simulink model "summary"  (R2022b)
settings: Solver=FixedStepAuto  StartTime=0.0  StopTime=20  FixedStep=0.1  RelTol=1e-3
values from neighbouring files (symbols this model uses):
  C_M = 1.1366    [MPC.m]
  C_T = 3.5611    [MPC.m]
  D_p = 0.1    [MPC.m]
  disturbance_f = 10    [MPC.m]    (also in generate_disturbance.m = f_min   + (f_max - f_min)   * rand(N, 1))
  disturbance_tau_x = 0.1    [MPC.m]    (also in generate_disturbance.m = tau_min + (tau_max - tau_min) * rand(N, 1))
  disturbance_tau_y = 0    [MPC.m]    (also in generate_disturbance.m = tau_min + (tau_max - tau_min) * rand(N, 1))
  disturbance_tau_z = 0    [MPC.m]    (also in generate_disturbance.m = tau_min + (tau_max - tau_min) * rand(N, 1))
  f_max = 10    [MPC.m]    (also in generate_disturbance.m)
  ModelInit_Att_x = 0    [MPC.m]
  ModelInit_Att_y = 0    [MPC.m]
  ModelInit_Att_z = 0    [MPC.m]
  ModelInit_Pos_x = 0    [MPC.m]
  ModelInit_Pos_y = 0    [MPC.m]
  ModelInit_Pos_z = 0    [MPC.m]
  ModelParam_c_M = 1.779e-07*2    (= 3.558e-07)    [MPC.m]
  ModelParam_c_T = 1.105e-05    [MPC.m]
  ModelParam_d = 0.225    [MPC.m]
  ModelParam_g = 9.8    [MPC.m]
  ModelParam_I_xx = 0.0211    [MPC.m]
  ModelParam_I_yy = 0.0219    [MPC.m]
  ModelParam_I_zz = 0.0366    [MPC.m]
  ModelParam_J_RP = 0.0001287    [MPC.m]
  ModelParam_m = 1.4    [MPC.m]
  p = 1.225    [MPC.m]    (also in draw_real_and_posiblility.m = alpha_smooth * p + (1 - alpha_smooth) * p_prev)
  tau_max = 0.1    [MPC.m]    (also in generate_disturbance.m = 0.25)
libraries: mpclib x3
settings Model: Creator=12854  LastModifiedBy=12854
settings OptimizationCC: BlockReduction=off  DefaultParameterBehavior=Inlined  BufferReuse=off

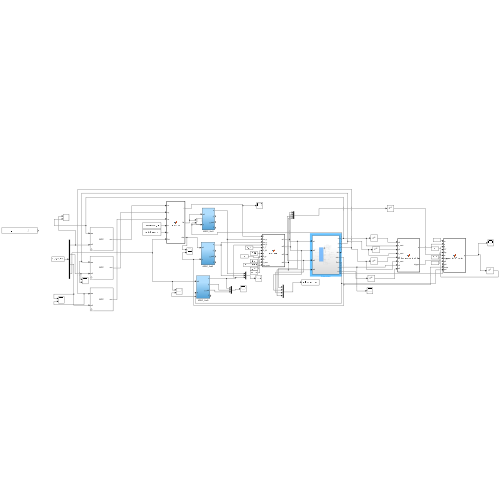
[thumbnail: Simulink's stored preview of the top-level diagram]
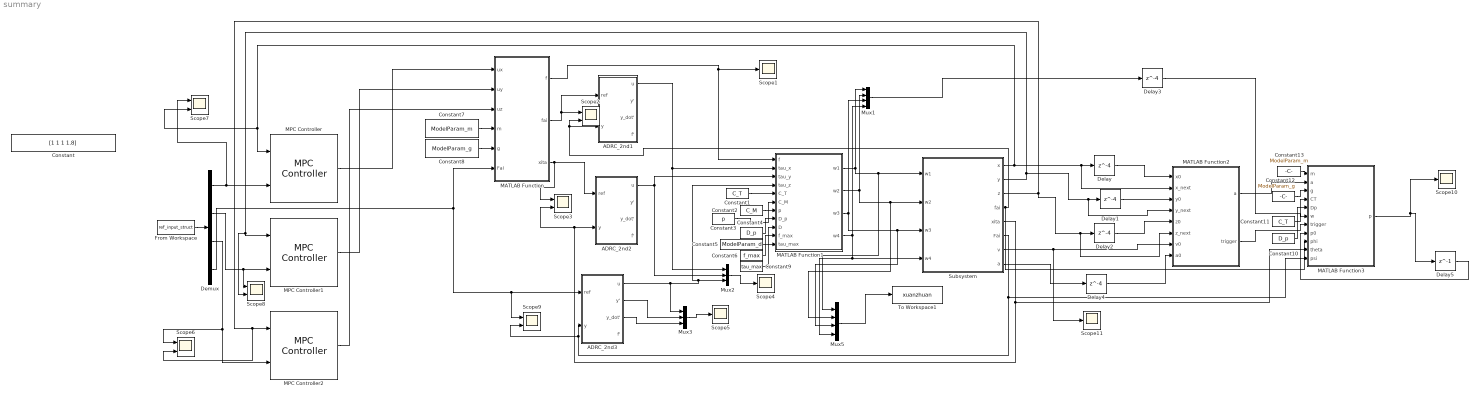
== system summary ==
  ADRC_2nd1 : Subsystem
  ADRC_2nd2 : Subsystem
  ADRC_2nd3 : Subsystem
  Constant : Constant  Value=[1 1 1 1.8]
  Constant1 : Constant  Value=C_T
  Constant10 : Constant  Value=D_p
  Constant11 : Constant  Value=C_T
  Constant12 : Constant  Value=ModelParam_g
  Constant13 : Constant  Value=ModelParam_m
  Constant2 : Constant  Value=C_M
  Constant3 : Constant  Value=p
  Constant4 : Constant  Value=D_p
  Constant5 : Constant  Value=ModelParam_d
  Constant6 : Constant  Value=f_max
  Constant7 : Constant  Value=ModelParam_m
  Constant8 : Constant  Value=ModelParam_g
  Constant9 : Constant  Value=tau_max
  Delay{,1..4} (5 alike) : Delay  DelayLength=4  InitialCondition=0
  Delay5 : Delay  DelayLength=1  InitialCondition=1.225
  Demux : Demux
  From Workspace : FromWorkspace  VariableName=ref_input_struct
  MATLAB Function : MATLAB Function  TreatAsAtomicUnit=on
  MATLAB Function1 : MATLAB Function  TreatAsAtomicUnit=on
  MATLAB Function2 : MATLAB Function  TreatAsAtomicUnit=on
  MATLAB Function3 : MATLAB Function  TreatAsAtomicUnit=on
  MPC Controller : mpclib/MPC Controller  SCDEnableBlockLinearizationSpecification=on  mpcobj=mpcobj_x  x0=[]  is_multiple=0  enable_value=0  return_u0=off  updateMPCinCallerWorkspace=on  md_inport=off  mv_inport=off  uref_inport=off  return_cost=off  return_mvseq=off  return_qpstatus=off  return_xseq=off  return_state=off  return_ovseq=off  state_inport=off  umin_inport=off  umax_inport=off  ymin_inport=off  ymax_inport=off  cc_inport=off  ywt_inport=off  uwt_inport=off  duwt_inport=off  rhoeps_inport=off  pm_inport=off  MaximumP=10  HorizonChoice=FixedHorizon  n_ts=0.1  n_p=10  n_mv=1  n_md=0  n_ud=0  n_mo=1  n_uo=0  BlockDataType=double  SampleTimeInherited=off  switch_inport=off
  MPC Controller1 : mpclib/MPC Controller  SCDEnableBlockLinearizationSpecification=on  mpcobj=mpcobj_y  x0=[]  is_multiple=0  enable_value=0  return_u0=off  updateMPCinCallerWorkspace=on  md_inport=off  mv_inport=off  uref_inport=off  return_cost=off  return_mvseq=off  return_qpstatus=off  return_xseq=off  return_state=off  return_ovseq=off  state_inport=off  umin_inport=off  umax_inport=off  ymin_inport=off  ymax_inport=off  cc_inport=off  ywt_inport=off  uwt_inport=off  duwt_inport=off  rhoeps_inport=off  pm_inport=off  MaximumP=10  HorizonChoice=FixedHorizon  n_ts=0.1  n_p=10  n_mv=1  n_md=0  n_ud=0  n_mo=1  n_uo=0  BlockDataType=double  SampleTimeInherited=off  switch_inport=off
  MPC Controller2 : mpclib/MPC Controller  SCDEnableBlockLinearizationSpecification=on  mpcobj=mpcobj_z  x0=[]  is_multiple=0  enable_value=0  return_u0=off  updateMPCinCallerWorkspace=on  md_inport=off  mv_inport=off  uref_inport=off  return_cost=off  return_mvseq=off  return_qpstatus=off  return_xseq=off  return_state=off  return_ovseq=off  state_inport=off  umin_inport=off  umax_inport=off  ymin_inport=off  ymax_inport=off  cc_inport=off  ywt_inport=off  uwt_inport=off  duwt_inport=off  rhoeps_inport=off  pm_inport=off  MaximumP=10  HorizonChoice=FixedHorizon  n_ts=0.1  n_p=10  n_mv=1  n_md=0  n_ud=0  n_mo=1  n_uo=0  BlockDataType=double  SampleTimeInherited=off  switch_inport=off
  Mux1 : Mux
  Mux2 : Mux  Inputs=3
  Mux3 : Mux  Inputs=3
  Mux5 : Mux
  Scope{1,4..5,10..11} (5 alike) : Scope
  Scope{2..3,6..9} (6 alike) : Scope  NumInputPorts=2
  Subsystem : Subsystem
  To Workspace1 : ToWorkspace  VariableName=xuanzhuan  SaveFormat=Timeseries  SampleTime=-1
  wires:
  Subsystem/1(x) -> MPC Controller/1, Scope7/2, MATLAB Function2/2(x_next), Delay/1
  Subsystem/2(y) -> Scope8/2, MPC Controller1/1, MATLAB Function2/4(y_next), Delay1/1
  Subsystem/3(z) -> MATLAB Function2/6(z_next), Delay2/1, Scope6/2, MPC Controller2/1
  Demux/1 -> Scope7/1, MPC Controller/2
  Demux/2 -> Scope8/1, MPC Controller1/2
  Demux/3 -> Scope6/1, MPC Controller2/2
  From Workspace/1 -> Demux/1
  MPC Controller/1 -> MATLAB Function/1(ux)
  MPC Controller1/1 -> MATLAB Function/2(uy)
  MPC Controller2/1 -> MATLAB Function/3(uz)
  Demux/4 -> Scope9/1, ADRC_2nd3/1(ref), MATLAB Function/6(Fai)
  Constant8/1 -> MATLAB Function/5(g)
  Constant7/1 -> MATLAB Function/4(m)
  MATLAB Function/1(f) -> Scope1/1, MATLAB Function1/1(f)
  Subsystem/4(fai) -> ADRC_2nd1/2(y), Scope2/2, MATLAB Function3/9(phi)
  MATLAB Function/2(fai) -> ADRC_2nd1/1(ref), Scope2/1
  MATLAB Function/3(xita) -> ADRC_2nd2/1(ref), Scope3/1
  Subsystem/5(xita) -> MATLAB Function3/10(theta), ADRC_2nd2/2(y), Scope3/2
  Subsystem/6(Fai) -> MATLAB Function3/11(psi), Scope9/2, ADRC_2nd3/2(y)
  ADRC_2nd3/1(u) -> Mux2/3, MATLAB Function1/4(tau_z), Mux3/1
  MATLAB Function1/1(w1) -> Mux1/1, Mux5/1, Subsystem/1(w1)
  MATLAB Function1/2(w2) -> Mux1/2, Mux5/2, Subsystem/2(w2)
  MATLAB Function1/3(w3) -> Mux1/3, Mux5/3, Subsystem/3(w3)
  MATLAB Function1/4(w4) -> Subsystem/4(w4), Mux5/4, Mux1/4
  Constant1/1 -> MATLAB Function1/5(C_T)
  Constant2/1 -> MATLAB Function1/6(C_M)
  Constant4/1 -> MATLAB Function1/8(D_p)
  Constant5/1 -> MATLAB Function1/9(D)
  Mux2/1 -> Scope4/1
  Constant6/1 -> MATLAB Function1/10(f_max)
  Constant9/1 -> MATLAB Function1/11(tau_max)
  Mux3/1 -> Scope5/1
  ADRC_2nd3/2(y') -> Mux3/2
  ADRC_2nd3/3(y_dot') -> Mux3/3
  ADRC_2nd1/1(u) -> Mux2/1, MATLAB Function1/2(tau_x)
  ADRC_2nd2/1(u) -> Mux2/2, MATLAB Function1/3(tau_y)
  Subsystem/7(v) -> Scope11/1, MATLAB Function2/7(v0)
  Delay/1 -> MATLAB Function2/1(x0)
  Delay1/1 -> MATLAB Function2/3(y0)
  Delay2/1 -> MATLAB Function2/5(z0)
  MATLAB Function2/1(a) -> MATLAB Function3/2(a)
  Constant10/1 -> MATLAB Function3/5(Dp)
  Constant11/1 -> MATLAB Function3/4(CT)
  Constant12/1 -> MATLAB Function3/3(g)
  Constant13/1 -> MATLAB Function3/1(m)
  Mux1/1 -> Delay3/1
  Delay3/1 -> MATLAB Function3/6(w)
  Subsystem/8(a) -> Delay4/1
  Delay4/1 -> MATLAB Function2/8(a0)
  MATLAB Function2/2(trigger) -> MATLAB Function3/7(trigger)
  Delay5/1 -> MATLAB Function3/8(p0)
  Constant3/1 -> MATLAB Function1/7(p)
  MATLAB Function3/1(p) -> Scope10/1, Delay5/1
  Mux5/1 -> To Workspace1/1

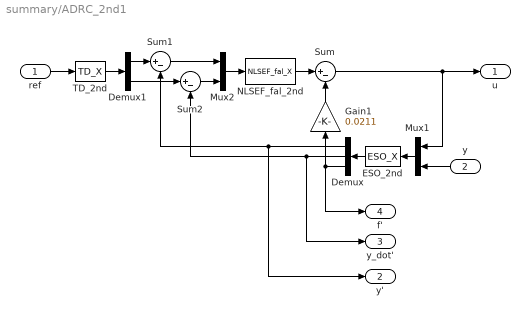
== system summary/ADRC_2nd1 ==
  ref : Inport
  y : Inport  Port=2
  Demux : Demux  Outputs=3
  Demux1 : Demux  Outputs=2
  ESO_2nd : S-Function  FunctionName=ESO_X  Parameters=CtrlParaX  SFunctionDeploymentMode=off  EnableBusSupport=off
  Gain1 : Gain  Gain=0.0211
  Mux1 : Mux  Inputs=2
  Mux2 : Mux  Inputs=2
  NLSEF_fal_2nd : S-Function  FunctionName=NLSEF_fal_X  Parameters=CtrlParaX  SFunctionDeploymentMode=off  EnableBusSupport=off
  Sum : Sum  Inputs=|+-
  Sum1 : Sum  Inputs=|+-
  Sum2 : Sum  Inputs=|+-
  TD_2nd : S-Function  FunctionName=TD_X  Parameters=CtrlParaX  SFunctionDeploymentMode=off  EnableBusSupport=off
  u : Outport  VectorParamsAs1DForOutWhenUnconnected=off
  y' : Outport  Port=2  VectorParamsAs1DForOutWhenUnconnected=off
  y_dot' : Outport  Port=3  VectorParamsAs1DForOutWhenUnconnected=off
  f' : Outport  Port=4  VectorParamsAs1DForOutWhenUnconnected=off
  wires:
  Mux2/1 -> NLSEF_fal_2nd/1
  ESO_2nd/1 -> Demux/1
  Demux1/2 -> Sum2/1
  ref/1 -> TD_2nd/1
  Demux/1 -> y'/1, Sum1/2
  TD_2nd/1 -> Demux1/1
  y/1 -> Mux1/2
  Gain1/1 -> Sum/2
  Demux/2 -> y_dot'/1, Sum2/2
  Demux1/1 -> Sum1/1
  Demux/3 -> Gain1/1, f'/1
  Sum2/1 -> Mux2/2
  Sum/1 -> Mux1/1, u/1
  NLSEF_fal_2nd/1 -> Sum/1
  Sum1/1 -> Mux2/1
  Mux1/1 -> ESO_2nd/1

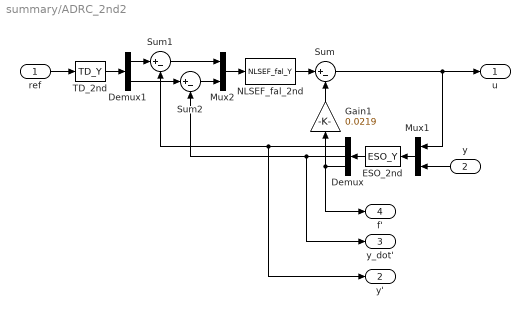
== system summary/ADRC_2nd2 ==
  ref : Inport
  y : Inport  Port=2
  Demux : Demux  Outputs=3
  Demux1 : Demux  Outputs=2
  ESO_2nd : S-Function  FunctionName=ESO_Y  Parameters=CtrlParaY  SFunctionDeploymentMode=off  EnableBusSupport=off
  Gain1 : Gain  Gain=0.0219
  Mux1 : Mux  Inputs=2
  Mux2 : Mux  Inputs=2
  NLSEF_fal_2nd : S-Function  FunctionName=NLSEF_fal_Y  Parameters=CtrlParaY  SFunctionDeploymentMode=off  EnableBusSupport=off
  Sum : Sum  Inputs=|+-
  Sum1 : Sum  Inputs=|+-
  Sum2 : Sum  Inputs=|+-
  TD_2nd : S-Function  FunctionName=TD_Y  Parameters=CtrlParaY  SFunctionDeploymentMode=off  EnableBusSupport=off
  u : Outport  VectorParamsAs1DForOutWhenUnconnected=off
  y' : Outport  Port=2  VectorParamsAs1DForOutWhenUnconnected=off
  y_dot' : Outport  Port=3  VectorParamsAs1DForOutWhenUnconnected=off
  f' : Outport  Port=4  VectorParamsAs1DForOutWhenUnconnected=off
  wires:
  Mux2/1 -> NLSEF_fal_2nd/1
  ESO_2nd/1 -> Demux/1
  Demux1/2 -> Sum2/1
  ref/1 -> TD_2nd/1
  Demux/1 -> y'/1, Sum1/2
  TD_2nd/1 -> Demux1/1
  y/1 -> Mux1/2
  Gain1/1 -> Sum/2
  Demux/2 -> y_dot'/1, Sum2/2
  Demux1/1 -> Sum1/1
  Demux/3 -> Gain1/1, f'/1
  Sum2/1 -> Mux2/2
  Sum/1 -> Mux1/1, u/1
  NLSEF_fal_2nd/1 -> Sum/1
  Sum1/1 -> Mux2/1
  Mux1/1 -> ESO_2nd/1

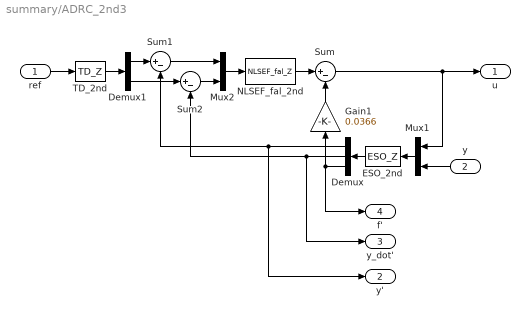
== system summary/ADRC_2nd3 ==
  ref : Inport
  y : Inport  Port=2
  Demux : Demux  Outputs=3
  Demux1 : Demux  Outputs=2
  ESO_2nd : S-Function  FunctionName=ESO_Z  Parameters=CtrlParaZ  SFunctionDeploymentMode=off  EnableBusSupport=off
  Gain1 : Gain  Gain=0.0366
  Mux1 : Mux  Inputs=2
  Mux2 : Mux  Inputs=2
  NLSEF_fal_2nd : S-Function  FunctionName=NLSEF_fal_Z  Parameters=CtrlParaZ  SFunctionDeploymentMode=off  EnableBusSupport=off
  Sum : Sum  Inputs=|+-
  Sum1 : Sum  Inputs=|+-
  Sum2 : Sum  Inputs=|+-
  TD_2nd : S-Function  FunctionName=TD_Z  Parameters=CtrlParaZ  SFunctionDeploymentMode=off  EnableBusSupport=off
  u : Outport  VectorParamsAs1DForOutWhenUnconnected=off
  y' : Outport  Port=2  VectorParamsAs1DForOutWhenUnconnected=off
  y_dot' : Outport  Port=3  VectorParamsAs1DForOutWhenUnconnected=off
  f' : Outport  Port=4  VectorParamsAs1DForOutWhenUnconnected=off
  wires:
  Mux2/1 -> NLSEF_fal_2nd/1
  ESO_2nd/1 -> Demux/1
  Demux1/2 -> Sum2/1
  ref/1 -> TD_2nd/1
  Demux/1 -> y'/1, Sum1/2
  TD_2nd/1 -> Demux1/1
  y/1 -> Mux1/2
  Gain1/1 -> Sum/2
  Demux/2 -> y_dot'/1, Sum2/2
  Demux1/1 -> Sum1/1
  Demux/3 -> Gain1/1, f'/1
  Sum2/1 -> Mux2/2
  Sum/1 -> Mux1/1, u/1
  NLSEF_fal_2nd/1 -> Sum/1
  Sum1/1 -> Mux2/1
  Mux1/1 -> ESO_2nd/1

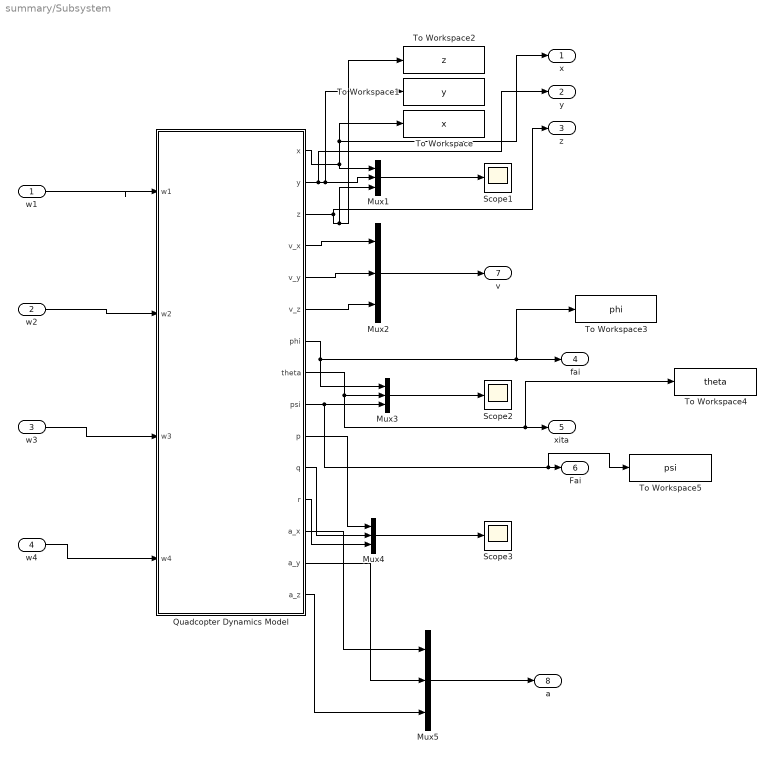
== system summary/Subsystem ==
  w1 : Inport
  w2 : Inport  Port=2
  w3 : Inport  Port=3
  w4 : Inport  Port=4
  Mux{1..5} (5 alike) : Mux  Inputs=3
  Quadcopter Dynamics Model : Subsystem
  Scope1 : Scope
  Scope2 : Scope
  Scope3 : Scope
  To Workspace : ToWorkspace  VariableName=x  SaveFormat=Timeseries  SampleTime=-1
  To Workspace1 : ToWorkspace  VariableName=y  SaveFormat=Timeseries  SampleTime=-1
  To Workspace2 : ToWorkspace  VariableName=z  SaveFormat=Timeseries  SampleTime=-1
  To Workspace3 : ToWorkspace  VariableName=phi  SaveFormat=Timeseries  SampleTime=-1
  To Workspace4 : ToWorkspace  VariableName=theta  SaveFormat=Timeseries  SampleTime=-1
  To Workspace5 : ToWorkspace  VariableName=psi  SaveFormat=Timeseries  SampleTime=-1
  x : Outport
  y : Outport  Port=2
  z : Outport  Port=3
  fai : Outport  Port=4
  xita : Outport  Port=5
  Fai : Outport  Port=6
  v : Outport  Port=7
  a : Outport  Port=8
  wires:
  Mux4/1 -> Scope3/1
  Mux3/1 -> Scope2/1
  Quadcopter Dynamics Model/2(y) -> y/1, To Workspace1/1, Mux1/2
  Quadcopter Dynamics Model/8(theta) -> To Workspace4/1, xita/1, Mux3/2
  Quadcopter Dynamics Model/5(v_y) -> Mux2/2
  Quadcopter Dynamics Model/1(x) -> x/1, To Workspace/1, Mux1/1
  Quadcopter Dynamics Model/6(v_z) -> Mux2/3
  Mux2/1 -> v/1
  Quadcopter Dynamics Model/12(r) -> Mux4/3
  Mux1/1 -> Scope1/1
  Quadcopter Dynamics Model/10(p) -> Mux4/1
  Quadcopter Dynamics Model/4(v_x) -> Mux2/1
  Quadcopter Dynamics Model/7(phi) -> Mux3/1, To Workspace3/1, fai/1
  Quadcopter Dynamics Model/3(z) -> To Workspace2/1, Mux1/3, z/1
  Quadcopter Dynamics Model/11(q) -> Mux4/2
  Quadcopter Dynamics Model/9(psi) -> To Workspace5/1, Fai/1, Mux3/3
  w1/1 -> Quadcopter Dynamics Model/1(w1)
  w2/1 -> Quadcopter Dynamics Model/2(w2)
  w3/1 -> Quadcopter Dynamics Model/3(w3)
  w4/1 -> Quadcopter Dynamics Model/4(w4)
  Quadcopter Dynamics Model/15(a_z) -> Mux5/3
  Quadcopter Dynamics Model/14(a_y) -> Mux5/2
  Quadcopter Dynamics Model/13(a_x) -> Mux5/1
  Mux5/1 -> a/1

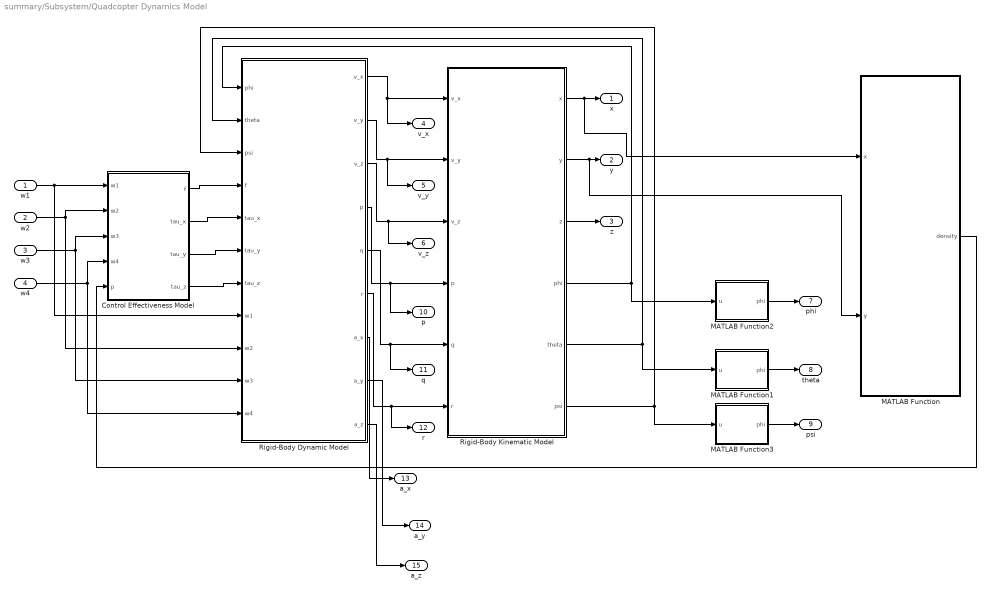
== system summary/Subsystem/Quadcopter Dynamics Model ==
  w1 : Inport
  w2 : Inport  Port=2
  w3 : Inport  Port=3
  w4 : Inport  Port=4
  Control Effectiveness Model : Subsystem
  MATLAB Function : MATLAB Function  TreatAsAtomicUnit=on
  MATLAB Function1 : MATLAB Function  TreatAsAtomicUnit=on
  MATLAB Function2 : MATLAB Function  TreatAsAtomicUnit=on
  MATLAB Function3 : MATLAB Function  TreatAsAtomicUnit=on
  Rigid-Body Dynamic Model : Subsystem
  Rigid-Body Kinematic Model : Subsystem
  x : Outport  VectorParamsAs1DForOutWhenUnconnected=off
  y : Outport  Port=2  VectorParamsAs1DForOutWhenUnconnected=off
  z : Outport  Port=3  VectorParamsAs1DForOutWhenUnconnected=off
  v_x : Outport  Port=4  VectorParamsAs1DForOutWhenUnconnected=off
  v_y : Outport  Port=5  VectorParamsAs1DForOutWhenUnconnected=off
  v_z : Outport  Port=6  VectorParamsAs1DForOutWhenUnconnected=off
  phi : Outport  Port=7  VectorParamsAs1DForOutWhenUnconnected=off
  theta : Outport  Port=8  VectorParamsAs1DForOutWhenUnconnected=off
  psi : Outport  Port=9  VectorParamsAs1DForOutWhenUnconnected=off
  p : Outport  Port=10  VectorParamsAs1DForOutWhenUnconnected=off
  q : Outport  Port=11  VectorParamsAs1DForOutWhenUnconnected=off
  r : Outport  Port=12  VectorParamsAs1DForOutWhenUnconnected=off
  a_x : Outport  Port=13  VectorParamsAs1DForOutWhenUnconnected=off
  a_y : Outport  Port=14  VectorParamsAs1DForOutWhenUnconnected=off
  a_z : Outport  Port=15  VectorParamsAs1DForOutWhenUnconnected=off
  wires:
  w1/1 -> Rigid-Body Dynamic Model/8(w1), Control Effectiveness Model/1(w1)
  Control Effectiveness Model/1(f) -> Rigid-Body Dynamic Model/4(f)
  w3/1 -> Rigid-Body Dynamic Model/10(w3), Control Effectiveness Model/3(w3)
  w4/1 -> Rigid-Body Dynamic Model/11(w4), Control Effectiveness Model/4(w4)
  w2/1 -> Rigid-Body Dynamic Model/9(w2), Control Effectiveness Model/2(w2)
  Rigid-Body Dynamic Model/4(p) -> Rigid-Body Kinematic Model/4(p), p/1
  Rigid-Body Dynamic Model/3(v_z) -> Rigid-Body Kinematic Model/3(v_z), v_z/1
  Rigid-Body Dynamic Model/6(r) -> Rigid-Body Kinematic Model/6(r), r/1
  Control Effectiveness Model/2(tau_x) -> Rigid-Body Dynamic Model/5(tau_x)
  Rigid-Body Dynamic Model/2(v_y) -> Rigid-Body Kinematic Model/2(v_y), v_y/1
  Rigid-Body Kinematic Model/1(x) -> MATLAB Function/1(x), x/1
  Rigid-Body Dynamic Model/5(q) -> Rigid-Body Kinematic Model/5(q), q/1
  Control Effectiveness Model/4(tau_z) -> Rigid-Body Dynamic Model/7(tau_z)
  Rigid-Body Kinematic Model/2(y) -> MATLAB Function/2(y), y/1
  Rigid-Body Kinematic Model/3(z) -> z/1
  Rigid-Body Dynamic Model/1(v_x) -> v_x/1, Rigid-Body Kinematic Model/1(v_x)
  Control Effectiveness Model/3(tau_y) -> Rigid-Body Dynamic Model/6(tau_y)
  Rigid-Body Kinematic Model/4(phi) -> MATLAB Function2/1(u), Rigid-Body Dynamic Model/1(phi)
  Rigid-Body Kinematic Model/5(theta) -> MATLAB Function1/1(u), Rigid-Body Dynamic Model/2(theta)
  Rigid-Body Kinematic Model/6(psi) -> MATLAB Function3/1(u), Rigid-Body Dynamic Model/3(psi)
  MATLAB Function2/1(phi) -> phi/1
  MATLAB Function1/1(phi) -> theta/1
  MATLAB Function3/1(phi) -> psi/1
  MATLAB Function/1(density) -> Control Effectiveness Model/5(p)
  Rigid-Body Dynamic Model/7(a_x) -> a_x/1
  Rigid-Body Dynamic Model/8(a_y) -> a_y/1
  Rigid-Body Dynamic Model/9(a_z) -> a_z/1

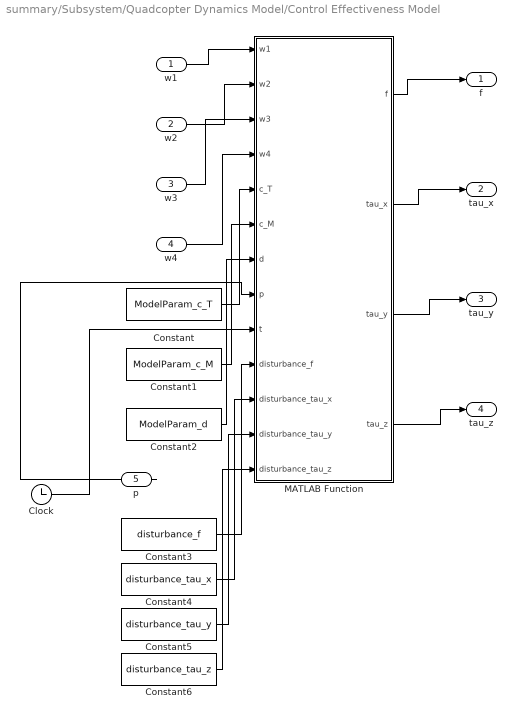
== system summary/Subsystem/Quadcopter Dynamics Model/Control Effectiveness Model ==
  w1 : Inport
  w2 : Inport  Port=2
  w3 : Inport  Port=3
  w4 : Inport  Port=4
  p : Inport  Port=5
  Clock : Clock
  Constant : Constant  Value=ModelParam_c_T
  Constant1 : Constant  Value=ModelParam_c_M
  Constant2 : Constant  Value=ModelParam_d
  Constant3 : Constant  Value=disturbance_f
  Constant4 : Constant  Value=disturbance_tau_x
  Constant5 : Constant  Value=disturbance_tau_y
  Constant6 : Constant  Value=disturbance_tau_z
  MATLAB Function : MATLAB Function  TreatAsAtomicUnit=on
  f : Outport  VectorParamsAs1DForOutWhenUnconnected=off
  tau_x : Outport  Port=2  VectorParamsAs1DForOutWhenUnconnected=off
  tau_y : Outport  Port=3  VectorParamsAs1DForOutWhenUnconnected=off
  tau_z : Outport  Port=4  VectorParamsAs1DForOutWhenUnconnected=off
  wires:
  Constant1/1 -> MATLAB Function/6(c_M)
  Constant/1 -> MATLAB Function/5(c_T)
  MATLAB Function/3(tau_y) -> tau_y/1
  MATLAB Function/1(f) -> f/1
  Constant2/1 -> MATLAB Function/7(d)
  MATLAB Function/4(tau_z) -> tau_z/1
  w3/1 -> MATLAB Function/3(w3)
  w1/1 -> MATLAB Function/1(w1)
  w4/1 -> MATLAB Function/4(w4)
  MATLAB Function/2(tau_x) -> tau_x/1
  w2/1 -> MATLAB Function/2(w2)
  p/1 -> MATLAB Function/8(p)
  Clock/1 -> MATLAB Function/9(t)
  Constant3/1 -> MATLAB Function/10(disturbance_f)
  Constant4/1 -> MATLAB Function/11(disturbance_tau_x)
  Constant5/1 -> MATLAB Function/12(disturbance_tau_y)
  Constant6/1 -> MATLAB Function/13(disturbance_tau_z)

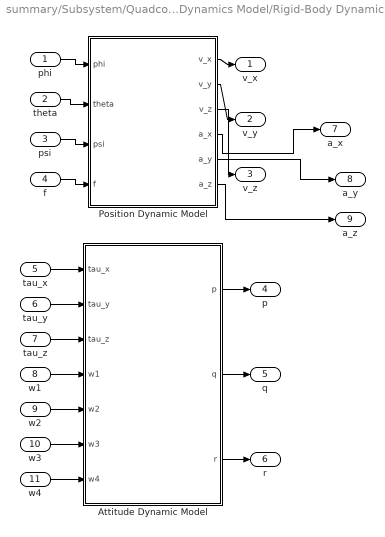
== system summary/Subsystem/Quadcopter Dynamics Model/Rigid-Body Dynamic Model ==
  phi : Inport
  theta : Inport  Port=2
  psi : Inport  Port=3
  f : Inport  Port=4
  tau_x : Inport  Port=5
  tau_y : Inport  Port=6
  tau_z : Inport  Port=7
  w1 : Inport  Port=8
  w2 : Inport  Port=9
  w3 : Inport  Port=10
  w4 : Inport  Port=11
  Attitude Dynamic Model : Subsystem
  Position Dynamic Model : Subsystem
  v_x : Outport  VectorParamsAs1DForOutWhenUnconnected=off
  v_y : Outport  Port=2  VectorParamsAs1DForOutWhenUnconnected=off
  v_z : Outport  Port=3  VectorParamsAs1DForOutWhenUnconnected=off
  p : Outport  Port=4  VectorParamsAs1DForOutWhenUnconnected=off
  q : Outport  Port=5  VectorParamsAs1DForOutWhenUnconnected=off
  r : Outport  Port=6  VectorParamsAs1DForOutWhenUnconnected=off
  a_x : Outport  Port=7  VectorParamsAs1DForOutWhenUnconnected=off
  a_y : Outport  Port=8  VectorParamsAs1DForOutWhenUnconnected=off
  a_z : Outport  Port=9  VectorParamsAs1DForOutWhenUnconnected=off
  wires:
  w3/1 -> Attitude Dynamic Model/6(w3)
  w1/1 -> Attitude Dynamic Model/4(w1)
  theta/1 -> Position Dynamic Model/2(theta)
  f/1 -> Position Dynamic Model/4(f)
  tau_x/1 -> Attitude Dynamic Model/1(tau_x)
  w2/1 -> Attitude Dynamic Model/5(w2)
  Attitude Dynamic Model/1(p) -> p/1
  w4/1 -> Attitude Dynamic Model/7(w4)
  Attitude Dynamic Model/2(q) -> q/1
  tau_y/1 -> Attitude Dynamic Model/2(tau_y)
  tau_z/1 -> Attitude Dynamic Model/3(tau_z)
  Position Dynamic Model/3(v_z) -> v_z/1
  Attitude Dynamic Model/3(r) -> r/1
  phi/1 -> Position Dynamic Model/1(phi)
  psi/1 -> Position Dynamic Model/3(psi)
  Position Dynamic Model/1(v_x) -> v_x/1
  Position Dynamic Model/2(v_y) -> v_y/1
  Position Dynamic Model/4(a_x) -> a_x/1
  Position Dynamic Model/5(a_y) -> a_y/1
  Position Dynamic Model/6(a_z) -> a_z/1

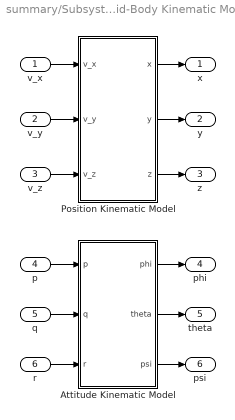
== system summary/Subsystem/Quadcopter Dynamics Model/Rigid-Body Kinematic Model ==
  v_x : Inport
  v_y : Inport  Port=2
  v_z : Inport  Port=3
  p : Inport  Port=4
  q : Inport  Port=5
  r : Inport  Port=6
  Attitude Kinematic Model : Subsystem
  Position Kinematic Model : Subsystem
  x : Outport  VectorParamsAs1DForOutWhenUnconnected=off
  y : Outport  Port=2  VectorParamsAs1DForOutWhenUnconnected=off
  z : Outport  Port=3  VectorParamsAs1DForOutWhenUnconnected=off
  phi : Outport  Port=4  VectorParamsAs1DForOutWhenUnconnected=off
  theta : Outport  Port=5  VectorParamsAs1DForOutWhenUnconnected=off
  psi : Outport  Port=6  VectorParamsAs1DForOutWhenUnconnected=off
  wires:
  v_x/1 -> Position Kinematic Model/1(v_x)
  v_y/1 -> Position Kinematic Model/2(v_y)
  r/1 -> Attitude Kinematic Model/3(r)
  p/1 -> Attitude Kinematic Model/1(p)
  v_z/1 -> Position Kinematic Model/3(v_z)
  Position Kinematic Model/1(x) -> x/1
  Position Kinematic Model/2(y) -> y/1
  q/1 -> Attitude Kinematic Model/2(q)
  Position Kinematic Model/3(z) -> z/1
  Attitude Kinematic Model/2(theta) -> theta/1
  Attitude Kinematic Model/1(phi) -> phi/1
  Attitude Kinematic Model/3(psi) -> psi/1

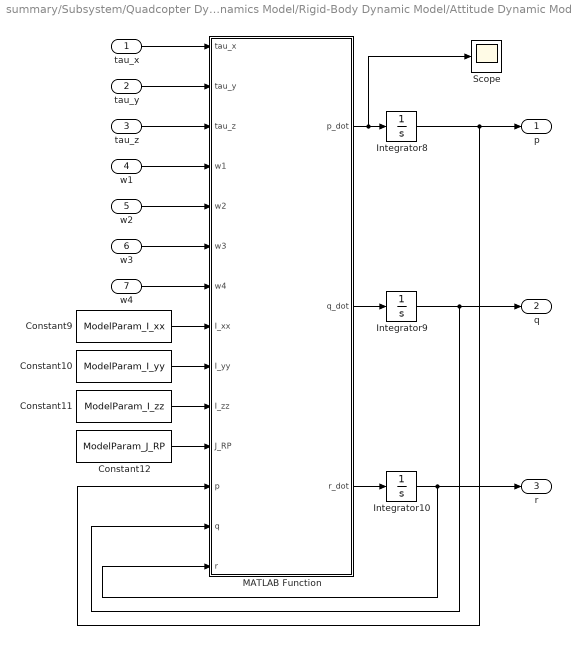
== system summary/Subsystem/Quadcopter Dynamics Model/Rigid-Body Dynamic Model/Attitude Dynamic Model ==
  tau_x : Inport
  tau_y : Inport  Port=2
  tau_z : Inport  Port=3
  w1 : Inport  Port=4
  w2 : Inport  Port=5
  w3 : Inport  Port=6
  w4 : Inport  Port=7
  Constant10 : Constant  Value=ModelParam_I_yy
  Constant11 : Constant  Value=ModelParam_I_zz
  Constant12 : Constant  Value=ModelParam_J_RP
  Constant9 : Constant  Value=ModelParam_I_xx
  Integrator10 : Integrator
  Integrator8 : Integrator
  Integrator9 : Integrator
  MATLAB Function : MATLAB Function  TreatAsAtomicUnit=on
  Scope : Scope
  p : Outport  VectorParamsAs1DForOutWhenUnconnected=off
  q : Outport  Port=2  VectorParamsAs1DForOutWhenUnconnected=off
  r : Outport  Port=3  VectorParamsAs1DForOutWhenUnconnected=off
  wires:
  Constant9/1 -> MATLAB Function/8(I_xx)
  tau_z/1 -> MATLAB Function/3(tau_z)
  Integrator10/1 -> r/1, MATLAB Function/14(r)
  Constant12/1 -> MATLAB Function/11(J_RP)
  Integrator9/1 -> q/1, MATLAB Function/13(q)
  Constant10/1 -> MATLAB Function/9(I_yy)
  MATLAB Function/3(r_dot) -> Integrator10/1
  MATLAB Function/1(p_dot) -> Scope/1, Integrator8/1
  Integrator8/1 -> p/1, MATLAB Function/12(p)
  tau_y/1 -> MATLAB Function/2(tau_y)
  MATLAB Function/2(q_dot) -> Integrator9/1
  Constant11/1 -> MATLAB Function/10(I_zz)
  w1/1 -> MATLAB Function/4(w1)
  tau_x/1 -> MATLAB Function/1(tau_x)
  w2/1 -> MATLAB Function/5(w2)
  w3/1 -> MATLAB Function/6(w3)
  w4/1 -> MATLAB Function/7(w4)

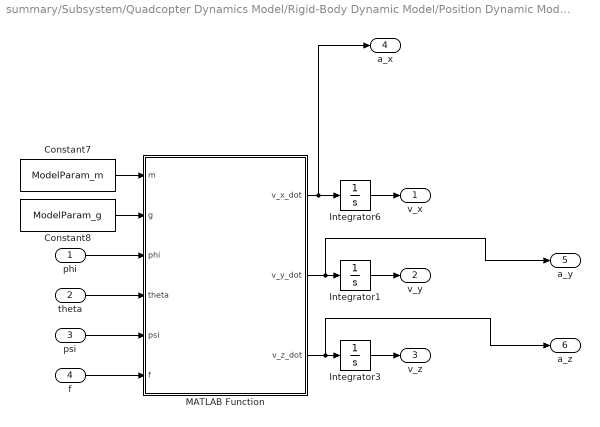
== system summary/Subsystem/Quadcopter Dynamics Model/Rigid-Body Dynamic Model/Position Dynamic Model ==
  phi : Inport
  theta : Inport  Port=2
  psi : Inport  Port=3
  f : Inport  Port=4
  Constant7 : Constant  Value=ModelParam_m
  Constant8 : Constant  Value=ModelParam_g
  Integrator1 : Integrator
  Integrator3 : Integrator
  Integrator6 : Integrator
  MATLAB Function : MATLAB Function  TreatAsAtomicUnit=on
  v_x : Outport  VectorParamsAs1DForOutWhenUnconnected=off
  v_y : Outport  Port=2  VectorParamsAs1DForOutWhenUnconnected=off
  v_z : Outport  Port=3  VectorParamsAs1DForOutWhenUnconnected=off
  a_x : Outport  Port=4  VectorParamsAs1DForOutWhenUnconnected=off
  a_y : Outport  Port=5  VectorParamsAs1DForOutWhenUnconnected=off
  a_z : Outport  Port=6  VectorParamsAs1DForOutWhenUnconnected=off
  wires:
  Constant8/1 -> MATLAB Function/2(g)
  MATLAB Function/1(v_x_dot) -> a_x/1, Integrator6/1
  MATLAB Function/2(v_y_dot) -> a_y/1, Integrator1/1
  theta/1 -> MATLAB Function/4(theta)
  Constant7/1 -> MATLAB Function/1(m)
  MATLAB Function/3(v_z_dot) -> a_z/1, Integrator3/1
  phi/1 -> MATLAB Function/3(phi)
  f/1 -> MATLAB Function/6(f)
  psi/1 -> MATLAB Function/5(psi)
  Integrator6/1 -> v_x/1
  Integrator1/1 -> v_y/1
  Integrator3/1 -> v_z/1

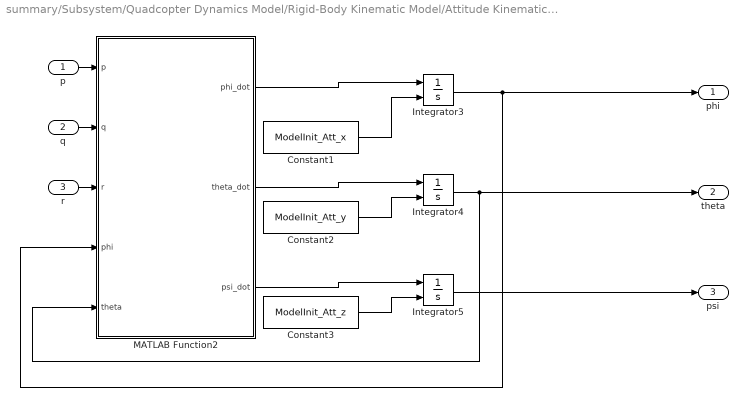
== system summary/Subsystem/Quadcopter Dynamics Model/Rigid-Body Kinematic Model/Attitude Kinematic Model ==
  p : Inport
  q : Inport  Port=2
  r : Inport  Port=3
  Constant1 : Constant  Value=ModelInit_Att_x
  Constant2 : Constant  Value=ModelInit_Att_y
  Constant3 : Constant  Value=ModelInit_Att_z
  Integrator3 : Integrator  InitialConditionSource=external
  Integrator4 : Integrator  InitialConditionSource=external
  Integrator5 : Integrator  InitialConditionSource=external
  MATLAB Function2 : MATLAB Function  TreatAsAtomicUnit=on
  phi : Outport  VectorParamsAs1DForOutWhenUnconnected=off
  theta : Outport  Port=2  VectorParamsAs1DForOutWhenUnconnected=off
  psi : Outport  Port=3  VectorParamsAs1DForOutWhenUnconnected=off
  wires:
  r/1 -> MATLAB Function2/3(r)
  MATLAB Function2/1(phi_dot) -> Integrator3/1
  q/1 -> MATLAB Function2/2(q)
  p/1 -> MATLAB Function2/1(p)
  MATLAB Function2/3(psi_dot) -> Integrator5/1
  MATLAB Function2/2(theta_dot) -> Integrator4/1
  Constant1/1 -> Integrator3/2
  Constant2/1 -> Integrator4/2
  Constant3/1 -> Integrator5/2
  Integrator3/1 -> phi/1, MATLAB Function2/4(phi)
  Integrator4/1 -> theta/1, MATLAB Function2/5(theta)
  Integrator5/1 -> psi/1

== system summary/Subsystem/Quadcopter Dynamics Model/Rigid-Body Kinematic Model/Position Kinematic Model ==
  v_x : Inport
  v_y : Inport  Port=2
  v_z : Inport  Port=3
  Constant1 : Constant  Value=ModelInit_Pos_z
  Constant2 : Constant  Value=ModelInit_Pos_y
  Constant3 : Constant  Value=ModelInit_Pos_x
  Integrator : Integrator  InitialConditionSource=external
  Integrator1 : Integrator  InitialConditionSource=external
  Integrator2 : Integrator  InitialConditionSource=external
  x : Outport  VectorParamsAs1DForOutWhenUnconnected=off
  y : Outport  Port=2  VectorParamsAs1DForOutWhenUnconnected=off
  z : Outport  Port=3  VectorParamsAs1DForOutWhenUnconnected=off
  wires:
  v_z/1 -> Integrator2/1
  Integrator1/1 -> y/1
  Integrator/1 -> x/1
  Constant1/1 -> Integrator2/2
  Integrator2/1 -> z/1
  v_x/1 -> Integrator/1
  v_y/1 -> Integrator1/1
  Constant2/1 -> Integrator1/2
  Constant3/1 -> Integrator/2

== matlab function summary/Subsystem/Quadcopter Dynamics Model/Rigid-Body Dynamic Model/Attitude Dynamic Model/MATLAB Function ==
  data: tau_x input; p_dot output; tau_y input; tau_z input; w1 input; w2 input; w3 input; w4 input; I_xx input; I_yy input; I_zz input; J_RP input; p input; q input; r input; q_dot output; r_dot output
function [p_dot, q_dot, r_dot] = fcn(tau_x, tau_y, tau_z, w1, w2, w3, w4, I_xx, I_yy, I_zz, J_RP, p, q, r)
% 函数描述
% 1.作用：本函数为四旋翼的姿态动力学微分方程组，通过四旋翼所受力矩和螺旋
%         桨转速计算得到四旋翼的机体角速度
% 2.函数输入：
%   wi：四个螺旋桨的转速(rad/s)
%   tau_x：x轴反扭力矩（机体轴）(N·m)
%   tau_y：y轴反扭力矩（机体轴）(N·m)
%   tau_z：z轴反扭力矩（机体轴）(N·m)
%   I_xx：四旋翼x轴转动惯量(kg·m^2)
%   I_yy：四旋翼y轴转动惯量(kg·m^2)
%   I_zz：四旋翼z轴转动惯量(kg·m^2)
%   J_RP：整个电机转子和螺旋桨绕转轴的总转动惯量(kg·m^2)
%   p：四旋翼x轴角速度（机体轴)(rad/s)
%   q：四旋翼y轴角速度（机体轴)(rad/s)
%   r：四旋翼z轴角速度（机体轴)(rad/s)
% 3.函数输出：
%   p_dot：四旋翼x轴角加速度（机体轴)
%   q_dot：四旋翼y轴角加速度（机体轴)
%   r_dot：四旋翼z轴角加速度（机体轴)
% 4.四旋翼构型为“X”型，螺旋桨序号如下所示：
%            1↑   2↓
%              \ /
%              / \
%            4↓   3↑
%   其中，↑表示螺旋桨逆时针旋转；↓表示螺旋桨顺时针旋转。

Omega = -w1 + w2 - w3 + w4;
p_dot = (1/I_xx) * (tau_x + q * r * (I_yy - I_zz) - J_RP * q * Omega);
q_dot = (1/I_yy) * (tau_y + p * r * (I_zz - I_xx) + J_RP * p * Omega);
r_dot = (1/I_zz) * (tau_z + p * q * (I_xx - I_yy) );
end

== matlab function summary/MATLAB Function1 ==
  data: f input; w1 output; tau_x input; tau_y input; w2 output; w3 output; tau_z input; w4 output; C_T input; C_M input; p input; D_p input; D input; f_max input; tau_max input
function [w1, w2, w3, w4] = converter(f, tau_x, tau_y, tau_z, C_T, C_M, p, D_p, D, f_max, tau_max)
%将推力和三轴转矩换算成电机转速
%需要的参数有 推力系数C_T、转矩系数C_M、空气密度ρ、螺旋桨直径D_p、无人机机臂长度D、最大推力f_max，最大转矩tau_max
%f = min(f, f_max);
%tau_x = min(tau_x, tau_max);
%tau_y = min(tau_y, tau_max);
%tau_z = min(tau_z, tau_max);
a = [f; tau_x; tau_y; tau_z];
A = [C_T*p*D_p^4/(4*pi^2), C_T*p*D_p^4/(4*pi^2), C_T*p*D_p^4/(4*pi^2), C_T*p*D_p^4/(4*pi^2); 
    sqrt(2)/2*D*C_T*p*D_p^4/(4*pi^2), -sqrt(2)/2*D*C_T*p*D_p^4/(4*pi^2), -sqrt(2)/2*D*C_T*p*D_p^4/(4*pi^2), sqrt(2)/2*D*C_T*p*D_p^4/(4*pi^2);
    sqrt(2)/2*D*C_T*p*D_p^4/(4*pi^2), sqrt(2)/2*D*C_T*p*D_p^4/(4*pi^2), -sqrt(2)/2*D*C_T*p*D_p^4/(4*pi^2), -sqrt(2)/2*D*C_T*p*D_p^4/(4*pi^2);
    C_M*p*D_p^5/(4*pi^2), -C_M*p*D_p^5/(4*pi^2), C_M*p*D_p^5/(4*pi^2), -C_M*p*D_p^5/(4*pi^2)];
%b = inv(A)*a;

b = A\a;

w12 = b(1);
w22 = b(2);
w32 = b(3);
w42 = b(4);

w12 = max(w12, 0);
w22 = max(w22, 0);
w32 = max(w32, 0);
w42 = max(w42, 0);

w1 = sqrt(w12);
w2 = sqrt(w22);
w3 = sqrt(w32);
w4 = sqrt(w42);
end

== matlab function summary/Subsystem/Quadcopter Dynamics Model/MATLAB Function1 ==
  data: u input; phi output
function phi  = fcn(u)

if u>0
    phi = mod(u,2*pi);

elseif u<0
    phi = mod(u,-2*pi);

else
    phi = 0;
end

== matlab function summary/Subsystem/Quadcopter Dynamics Model/MATLAB Function3 ==
  data: u input; phi output
function phi  = fcn(u)

if u>0
    phi = mod(u,2*pi);

elseif u<0
    phi = mod(u,-2*pi);

else
    phi = 0;
end

== matlab function summary/Subsystem/Quadcopter Dynamics Model/MATLAB Function ==
  data: x input; density output; y input
function density = air_density(x, y)
    % 定义火坑的中心位置
    center_x = 10;
    center_y = 10;

    % 定义火坑的半径
    radius = 3;

    % 定义火坑中心的空气密度为1.078 kg/m³
    density_center = 1.078;

    % 定义火坑边缘的空气密度为日常密度值
    density_edge = 1.225;

    % 计算无人机到火坑中心的距离
    r = sqrt((x - center_x)^2 + (y - center_y)^2);

    % 定义高斯函数的标准差
    sigma = radius / 3;
    
    % 使用高斯函数计算空气密度
    density = density_edge + (density_center - density_edge) * exp(-(r.^2) / (2 * sigma^2));


    density = density/1.225;
end

== matlab function summary/Subsystem/Quadcopter Dynamics Model/MATLAB Function2 ==
  data: u input; phi output
function phi  = fcn(u)

if u>0
    phi = mod(u,2*pi);

elseif u<0
    phi = mod(u,-2*pi);

else
    phi = 0;
end

== matlab function summary/MATLAB Function2 ==
  data: x0 input; a output; x_next input; y0 input; y_next input; z0 input; z_next input; v0 input; a0 input; trigger output
function [a,trigger]= calculateAccelerationPrime(x0, x_next, y0, y_next, z0, z_next, v0, a0)
Delta_t = 0.4;
P0 = [x0, y0, z0];
P1 = [x_next, y_next, z_next];

% 计算理论位置与实际位置的偏差
P = P0 + v0'.* Delta_t +a0./2.* Delta_t^2;
Delta_P_prime = P1 - P0 - v0' .* Delta_t;



% 根据位置偏差计算加速度
a = 2 * Delta_P_prime / (Delta_t^2);  % 计算实际加速度

distance = norm(P1 - P);

% 设置trigger条件
if distance > 0.7 && P1(1,3)>P(1,3)
    trigger = 1;
elseif distance <= 0.7 && P1(1,3) <= P(1,3) 
    trigger = 0;
else 
    trigger = 2;    
end
% 返回计算出的实际加速度

end

== matlab function summary/MATLAB Function3 ==
  data: m input; a input; p output; g input; CT input; Dp input; w input; trigger input; p0 input; phi input; theta input; psi input
function p = estimateAirDensity(m, a, g, CT, Dp, w, trigger, p0, phi, theta, psi)
    % m - 无人机质量
    % a - 实际测量的加速度向量 [ax, ay, az]
    % g - 重力加速度
    % CT - 推力系数  
    % Dp - 螺旋桨直径
    % w - 各螺旋桨的角速度数组 [w1; w2; w3; w4]
    p = 1.225;
    total_w2 = sum(w.^2);

    %p = (m .* a - m .* [0,0,g]') / (R * ((CT * Dp^4) .* [0, 0, total_w2]' ./ (4 * pi^2)));
    %v_x_dot = -f * (1/m) * (cos(psi) * sin(theta) * cos(phi) + sin(psi) * sin(phi));
    %v_y_dot = -f * (1/m) * (sin(psi) * sin(theta) * cos(phi) - cos(psi) * sin(phi));
    %v_z_dot = g - f * (1/m) * cos(phi) * cos(theta);

    if total_w2 > 0
        % 设置空气密度的初值
        %p = 1.225;  % 标准大气压下的空气密度，单位为kg/m³
        % 计算推力部分
        total_w2 = sum(w.^2)  % 计算所有螺旋桨的角速度平方和
        if trigger == 1
            % 假设 phi, theta, psi 是飞行器的欧拉角
        R = [cos(theta)*cos(psi), sin(phi)*sin(theta)*cos(psi) - cos(phi)*sin(psi), cos(phi)*sin(theta)*cos(psi) + sin(phi)*sin(psi);
                 cos(theta)*sin(psi), sin(phi)*sin(theta)*sin(psi) + cos(phi)*cos(psi), cos(phi)*sin(theta)*sin(psi) - sin(phi)*cos(psi);
                 -sin(theta),         sin(phi)*cos(theta),                             cos(phi)*cos(theta)];
        
        %p.*(R * ((CT * Dp^4) .* [0, 0, total_w2]' ./ (4 * pi^2))) = m .* a' - m .* [0,0,g]'  ;
        % 计算推力部分，即 T = R * (CT * Dp^4 * [0, 0, total_w2]' / (4 * pi^2))
        T = R * ((CT * Dp^4 * [0, 0, total_w2]' / (4 * pi^2)))
        
        % 计算外力 F = m * (a' - [0, 0, g]')
        F = m * (a' - [0, 0, g]')
    
        % 计算空气密度 p = norm(F) / norm(T)
        p = norm(F) / norm(T)
    
                
            % 计算空气密度
            %p = (m .* a - m .* [0,0,g]') / (R * ((CT * Dp^4) .* [0, 0, total_w2]' ./ (4 * pi^2)));
            %p = (m .* a - m .* [0,0,g]') / (R * ((CT * Dp^4) .* [0, 0, total_w2]' ./ (4 * pi^2)));
            %p = 1.225;
        else
            p = 1.225;
        end
    else
        p = 1.225;
    end
    
end

== matlab function summary/Subsystem/Quadcopter Dynamics Model/Rigid-Body Kinematic Model/Attitude Kinematic Model/MATLAB Function2 ==
  data: p input; phi_dot output; q input; r input; phi input; theta input; theta_dot output; psi_dot output
function [phi_dot, theta_dot, psi_dot] = fcn(p, q, r, phi, theta)
% 函数描述
% 1.作用：本函数为四旋翼的姿态运动学微分方程组，通过四旋翼的机体角速度
%         计算得到四旋翼的姿态角
% 2.函数输入：
%   p：四旋翼x轴角速度（机体轴)(rad/s)
%   q：四旋翼y轴角速度（机体轴)(rad/s)
%   r：四旋翼z轴角速度（机体轴)(rad/s)
%   phi：滚转角(rad)
%   theta：俯仰角(rad)
% 3.函数输出：
%   phi_dot：滚转角速度
%   theta_dot：俯仰角速度
%   psi_dot：偏航角速度
% 4.四旋翼构型为“X”型，螺旋桨序号如下所示：
%            3↓   1↑
%              \ /
%              / \
%            2↑   4↓
%   其中，↑表示螺旋桨逆时针旋转；↓表示螺旋桨顺时针旋转。

%大角度飞行
%phi_dot = p + q * tan(theta) * sin(phi) + r * tan(theta) * cos(phi);
%theta_dot = q * cos(phi) - r * sin(phi);
%psi_dot = (q * sin(phi) + r * cos(phi)) / cos(theta);

%小角度飞行
phi_dot = p;
theta_dot = q;
psi_dot = r;

end

== matlab function summary/Subsystem/Quadcopter Dynamics Model/Control Effectiveness Model/MATLAB Function ==
  data: w1 input; f output; w2 input; w3 input; w4 input; c_T input; c_M input; d input; tau_x output; tau_y output; tau_z output; p input; t input; disturbance_f input; disturbance_tau_x input; disturbance_tau_y input; disturbance_tau_z input
function [f, tau_x, tau_y, tau_z] = fcn(w1, w2, w3, w4, c_T, c_M, d, p, t, disturbance_f, disturbance_tau_x, disturbance_tau_y, disturbance_tau_z)
% 函数描述
% 1.作用：本函数用来计算螺旋桨旋转产生的总拉力和反扭力矩。
% 2.函数输入：
%   wi：四个螺旋桨的转速(rad/s)
%   c_T：螺旋桨拉力系数
%   c_M：螺旋桨转矩系数
%   d：机体中心和任一电机的距离(m)
% 3.函数输出：
%   f：螺旋桨拉力（机体轴）
%   tau_x：x轴反扭力矩（机体轴）
%   tau_y：y轴反扭力矩（机体轴）
%   tau_z：z轴反扭力矩（机体轴）
% 4.四旋翼构型为“X”型，螺旋桨序号如下所示：
%            1↑   2↓
%              \ /
%              / \
%            4↓   3↑
%   其中，↑表示螺旋桨逆时针旋转；↓表示螺旋桨顺时针旋转。

f = p*c_T * (w1^2 + w2^2 + w3^2 + w4^2);
tau_x = p*d * c_T * (sqrt(2)/2) * (w1^2 - w2^2 - w3^2 + w4^2);
tau_y = p*d * c_T * (sqrt(2)/2) * (w1^2 + w2^2 - w3^2 - w4^2);
tau_z = p*c_M * (w1^2 - w2^2 + w3^2 - w4^2);

% 添加扰动
if t == 5 % 在0.5s到0.6s之间添加扰动
    %disturbance_f = 1; % 拉力扰动量
    %disturbance_tau_x = 5; % tau_x扰动量
    %disturbance_tau_y = 0.0; % tau_x扰动量
    %disturbance_tau_z = 0.0; % tau_x扰动量
    f = f + disturbance_f;
    tau_x = tau_x + disturbance_tau_x;
    tau_y = tau_y + disturbance_tau_y;
    tau_z = tau_z + disturbance_tau_z;
end
end

== matlab function summary/MATLAB Function ==
  data: ux input; f output; uy input; uz input; fai output; xita output; m input; g input; Fai input
function [f, fai, xita] = converter(ux, uy, uz, m, g, Fai)
%将加速度ux uy uz换算成推力和参考滚转角、俯仰角
%需要的参数有 无人机质量m、重力加速度g、参考偏航角Fai
f = m * sqrt((ux)^2+uy^2+(uz-g)^2);
fai = asin((-m)/f*((ux)*sin(Fai)-uy*cos(Fai)));
xita = atan(1/(uz-g)*((ux)*cos(Fai)+uy*sin(Fai)));

end

== matlab function summary/Subsystem/Quadcopter Dynamics Model/Rigid-Body Dynamic Model/Position Dynamic Model/MATLAB Function ==
  data: m input; g input; phi input; theta input; psi input; f input; v_x_dot output; v_y_dot output; v_z_dot output
function [v_x_dot, v_y_dot, v_z_dot] = fcn(m, g, phi, theta, psi, f)
% 函数描述
% 1.作用：本函数为四旋翼的位置动力学微分方程组，通过四旋翼所受拉力、姿态角
%         计算得到四旋翼飞行器的加速度
% 2.函数输入：
%   m：四旋翼飞行器质量(kg)
%   g：重力加速度(m/s^2)
%   phi：滚转角(rad)
%   theta：俯仰角(rad)
%   psi：偏航角(rad)
%   f：螺旋桨产生的总拉力(N)
% 3.函数输出：
%   v_x_dot：地球坐标系下沿x轴的速度的导数
%   v_y_dot：地球坐标系下沿y轴的速度的导数
%   v_z_dot：地球坐标系下沿z轴的速度的导数
% 4.四旋翼构型为“X”型，螺旋桨序号如下所示：
%            3↓   1↑
%              \ /
%              / \
%            2↑   4↓
%   其中，↑表示螺旋桨逆时针旋转；↓表示螺旋桨顺时针旋转。

v_x_dot = -f * (1/m) * (cos(psi) * sin(theta) * cos(phi) + sin(psi) * sin(phi));
v_y_dot = -f * (1/m) * (sin(psi) * sin(theta) * cos(phi) - cos(psi) * sin(phi));
v_z_dot = g - f * (1/m) * cos(phi) * cos(theta);
end
